simulink model "AutofocusScene"  (R2026a)
settings: Solver=FixedStepDiscrete  StopTime=Cam_SweepTime + Cam_TailTime  FixedStep=Scene_Ts
model workspace (MAT data in the model file):
  AF_CoarseStep = 0.04
  AF_ConfirmTime = 0.25
  AF_FineSpan = 0.04
  AF_FineStep = 0.012
  AF_FocusMax = 30
  AF_FocusMin = 3
  AF_Gain = 0.9
  AF_LevelFloor = 1e-06
  AF_LockThreshold = 0.015
  AF_MaxSlew = 0.08
  AF_MinDwell = 1
  AF_MinSweepSteps = 4
  AF_PeakRatio = 3
  AF_ProbeSize = 0.002
  AF_SearchTrigger = 0.5
  AF_SpotFraction = 0.195
  AF_StopFraction = 0.7
  AF_TopFraction = 0.1
  AF_WinMargin = 1.15
  Cam_FocalLength = [554 554]
  Cam_HandAmount = 1
  Cam_Height = 1.5
  Cam_ImageSize = [480 640]
  Cam_OpticalCenter = [320 240]
  Cam_Pitch = 5
  Cam_SweepTime = 25
  Cam_TailPitch = 10
  Cam_TailTime = 6
  Cam_X = 2.5
  Cam_Y = -2
  Cam_YawStart = -75
  Cam_YawSweep = 100
  Depth_MaxRange = 30
  Scene_Ts = 0.05
undefined symbols (not defined in the file or in its folder): Sim3dSensor
libraries: slpidlib x1, simulink x1, sim3dcameralib x1, sim3dlib x1
settings Model: SimulationMode=accelerator  Creator=csaunder  LastModifiedBy=csaunder
settings DebuggingCC: MergeDetectMultiDrivingBlocksExec=error
settings ModelReferenceCC: PropagateSignalLabelsOutOfModel=on

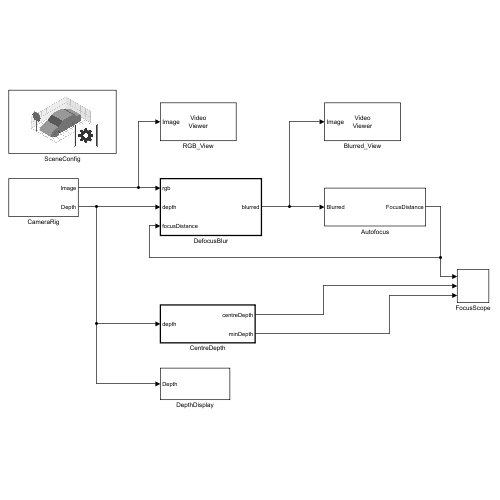
[thumbnail: Simulink's stored preview of the top-level diagram]
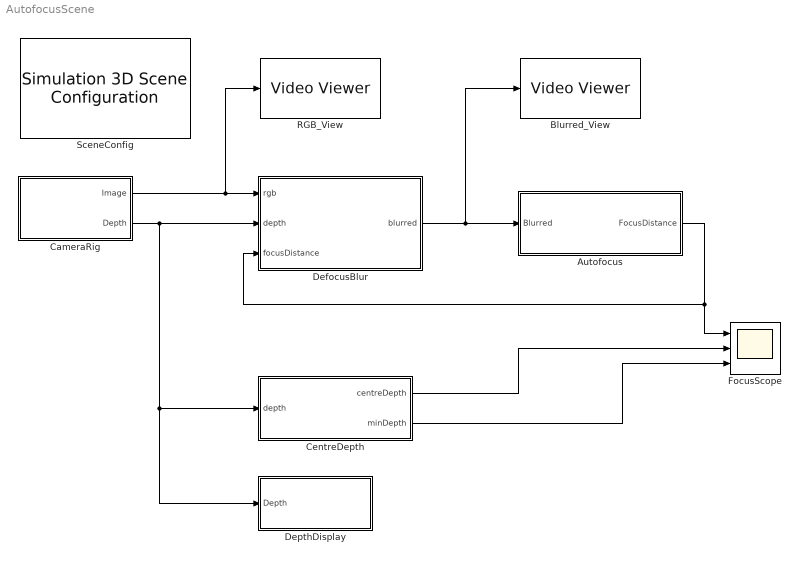
== system AutofocusScene ==
  Autofocus : Subsystem
  Blurred_View : VideoViewer  FigPos=[672 571 507 337]
  CameraRig : Subsystem
  CentreDepth : MATLAB Function  TreatAsAtomicUnit=on
  DefocusBlur : MATLAB Function  TreatAsAtomicUnit=on
  DepthDisplay : Subsystem
  FocusScope : Scope  NumInputPorts=3
  RGB_View : VideoViewer  FigPos=[99 545 418 304]
  SceneConfig : sim3dlib/Simulation 3D Scene Configuration  Priority=0  ProjectFormat=Default Scenes  SceneDesc=Large parking lot  ProjectName=C:\Program Files\MATLAB\R2026a\toolbox\shared\sim3d_projects\automotive_project_windows\UE\WindowsNoEditor\VehicleSimulation.exe  ScenePath=/Game/Maps/HwStrght  EnableOpenDRIVE=off  vehTagList={'Custom';'Scene Origin'}  vehTag=Scene Origin  AttachedCameraRelativeTranslation=[0 0 0]  FreeCameraDefaultInitialTranslation=[-6, 0, 2]  AttachedCameraRelativeRotation=[0, -15, 0]  FreeCameraDefaultInitialRotation=[0, -15, 0]  ViewpointName=Custom  FreeCameraInitialTranslation=[0, 0, 0]  FreeCameraInitialRotation=[0, 0, 0]  OpVisEn=off  Ts=Scene_Ts  EnableWindow=on  EnableRemoteAccess=off  SimulationMode=CoSimulation  SimulateUsing=Interpreted execution  EnableAnimationRecording=off  OverrideDefaultRecording=off  AnimationRecordingFileName=sim3dAnimation.mat  AnimationRecordingInterval=[0 inf]  EnableWeather=off  SunAzimuth=90  SunAltitude=40.0  EnableGeospatialSun=off  Latitude=0  Longitude=0  Date=2023-01-01  Time=10:30:00  GeoTimeZone=-5.0  SunDaylightSaving=off  wind=1  clouds=10  EnableVolumetricClouds=off  CloudCoverage=0  CloudAltitude=6  fog=0  rain=0  RaindropsEffect=off  SnowDensity=0  EnableGeospatial=off  TilesetSource=Earth terrain  UseTrueOrigin=off  OriginHeight=200  OriginLatitude=40.744652  OriginLongitude=-73.988864  MapStyle=Aerial  AdditionalAssetIDs=[]  UseAdvancedSunSky=off  SolarTime=11  TimeZone=-5  Day=21  Month=9  Year=2022  UseDaylightSavingTime=on  DSTStartDay=10  DSTStartMonth=3  DSTEndDay=3  DSTEndMonth=11  DSTSwitchHour=2  sensorTag=MainCamera1  sensorId=1  sensorName=MainCamera1  mountLoc=Origin  offsetFlag=off  tmountOffset=[0, 0, 0]  rmountOffset=[0, 0, 0]  HorizontalResolution=1280  VerticalResolution=720  HorizontalFOV=60  mountPoint=[0 0 0]  mountOrientation=[0 0 0]  aMode=5  ID=1  GeoTrigger=Inactive  ViewNameList={'Custom'}  ViewTranslationList={'[0 0 0]'}  ViewRotationList={'[0 0 0]'}
      link override Simulation 3D Engine: SceneDesc=Large parking lot
      settings: LibrarySourceBlock=sl3dlib/Simulation 3D/Environment/Simulation 3D Scene Configuration
  wires:
  CameraRig/1(Image) -> RGB_View/1, DefocusBlur/1(rgb)
  CameraRig/2(Depth) -> DepthDisplay/1(Depth), CentreDepth/1(depth), DefocusBlur/2(depth)
  DefocusBlur/1(blurred) -> Blurred_View/1, Autofocus/1(Blurred)
  Autofocus/1(FocusDistance) -> FocusScope/1, DefocusBlur/3(focusDistance)
  CentreDepth/1(centreDepth) -> FocusScope/2
  CentreDepth/2(minDepth) -> FocusScope/3

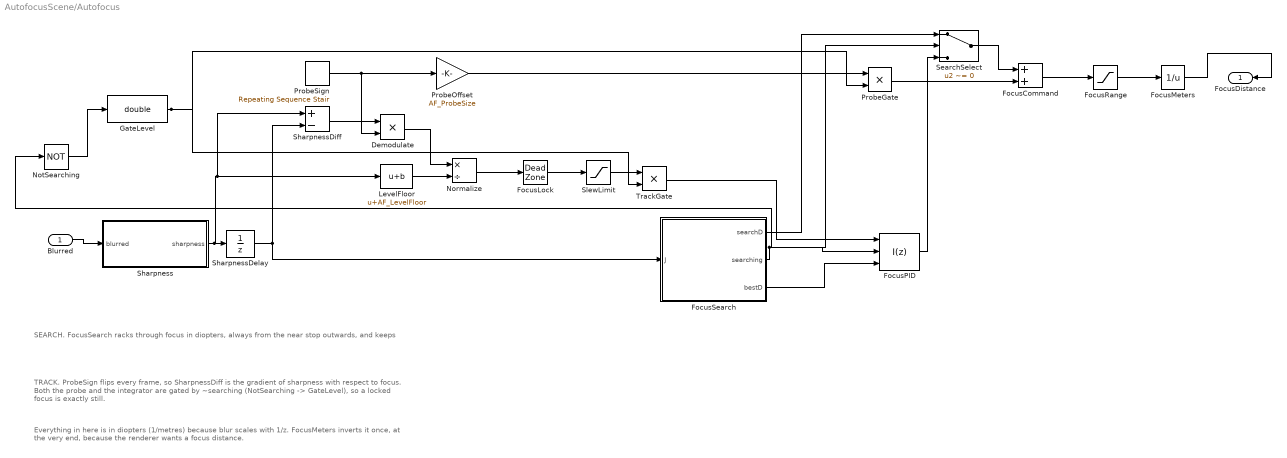
== system AutofocusScene/Autofocus ==
  note: SEARCH. FocusSearch racks through focus in diopters, always from the near stop outwards, and keeps
  note: TRACK. ProbeSign flips every frame, so SharpnessDiff is the gradient of sharpness with respect to focus.
      | Both the probe and the integrator are gated by ~searching (NotSearching -> GateLevel), so a locked focus is exactly still.
  note: Everything in here is in diopters (1/metres) because blur scales with 1/z. FocusMeters inverts it once, at the
      | very end, because the renderer wants a focus distance.
  Blurred : Inport
  Demodulate : Product
  FocusCommand : Sum
  FocusLock : DeadZone  LowerValue=-AF_LockThreshold  UpperValue=AF_LockThreshold
  FocusMeters : Math  Operator=reciprocal
  FocusPID : slpidlib/PID Controller  Controller=I  Form=Parallel  TimeDomain=Discrete-time  UseExternalTs=off  SampleTime=Scene_Ts  IntegratorMethod=Forward Euler  FilterMethod=Forward Euler  ControllerParametersSource=internal  P=1  I=AF_Gain  UseKiTs=off  D=0  UseExternalDerivativeSource=off  N=100  UseFilter=on  TunerSelectOption=Transfer Function Based (PID Tuner App)  InitialConditionSource=external  InitialConditionForIntegrator=1/10  InitialConditionForFilter=0  DifferentiatorICPrevScaledInput=0  ExternalReset=falling  TrackingMode=off  Kt=1  LimitOutput=on  SatLimitsSource=internal  UpperSaturationLimit=1/AF_FocusMin  LowerSaturationLimit=1/AF_FocusMax  LinearizeAsGain=on  AntiWindupMode=clamping  Kb=1  LimitIntegrator=off  UpperIntegratorSaturationLimit=inf  LowerIntegratorSaturationLimit=-inf  POutMin=[]  POutMax=[]  IOutMin=[]  IOutMax=[]  DOutMin=[]  DOutMax=[]  NOutMin=[]  NOutMax=[]  SumOutMin=[]  SumOutMax=[]  SaturationOutMin=[]  SaturationOutMax=[]  PParamMin=[]  PParamMax=[]  IParamMin=[]  IParamMax=[]  DParamMin=[]  DParamMax=[]  NParamMin=[]  NParamMax=[]  KbParamMin=[]  KbParamMax=[]  KtParamMin=[]  KtParamMax=[]  KbOutMin=[]  KbOutMax=[]  KtOutMin=[]  KtOutMax=[]  IntegratorOutMin=[]  IntegratorOutMax=[]  FilterOutMin=[]  FilterOutMax=[]  SumI1OutMin=[]  SumI1OutMax=[]  SumI2OutMin=[]  SumI2OutMax=[]  SumI3OutMin=[]  SumI3OutMax=[]  SumI4OutMin=[]  SumI4OutMax=[]  SumDOutMin=[]  SumDOutMax=[]  DifferentiatorOutMin=[]  DifferentiatorOutMax=[]  FilterDiffOutCoefMin=[]  FilterDiffOutCoefMax=[]  ReciprocalOutMin=[]  ReciprocalOutMax=[]  SumDenOutMin=[]  SumDenOutMax=[]  SumNumOutMin=[]  SumNumOutMax=[]  DivideOutMin=[]  DivideOutMax=[]  UdiffTsProdOutMin=[]  UdiffTsProdOutMax=[]  NTsProdOutMin=[]  NTsProdOutMax=[]  UintegralTsProdOutMin=[]  UintegralTsProdOutMax=[]  UngainTsProdOutMin=[]  UngainTsProdOutMax=[]  ClampingZeroOutDataTypeStr=Inherit: Inherit via back propagation  ClampingZeroOutMin=[]  ClampingZeroOutMax=[]  FilterDenConstantOutDataTypeStr=Inherit: Inherit via back propagation  FilterDenConstantOutMin=[]  FilterDenConstantOutMax=[]  PCopyOutDataTypeStr=Inherit: Inherit via back propagation  PCopyOutMin=[]  PCopyOutMax=[]  NCopyOutDataTypeStr=Inherit: Inherit via back propagation  NCopyOutMin=[]  NCopyOutMax=[]  IntegratorContinuousStateAttributes=''  IntegratorStateMustResolveToSignalObject=off  IntegratorRTWStateStorageClass=Auto  FilterContinuousStateAttributes=''  FilterStateMustResolveToSignalObject=off  FilterRTWStateStorageClass=Auto  ParallelPVariant=Disabled  IdealPVariant=Disabled  IVariant=InternalParameters  DVariant=Disabled  IntegratorVariant=Discrete  SatVariant=Enabled  AWVariant=DiscClampingParallel  PCopyVariant=Disabled  TRVariant=Disabled  FdbkBlocksVariant=Forward  IdealPFdbkVariant=Disabled  SatFdbkVariant=Disabled  DerivativeFilterVariant=Disabled  NVariant=Disabled  NCopyVariant=Disabled_SignalSpec  FilterICVariant=Disabled  IntegratorICVariant=ExternalICs  ExternalResetVariant=ExternalReset  TRSumVariant=Passthrough  SumFdbkVariant=Disabled  SumVariant=Passthrough_I  TsampFilterVariant=InternalTs  TsampNgainVariant=Passthrough  TsampIntegralVariant=Disabled_SignalSpec  ExternalSaturationOutDataTypeStr=Inherit: Same as second input  DerivativeSourceVariant=Disabled  PreIntVariant=InternalPreInt
  FocusRange : Saturate  UpperLimit=1/AF_FocusMin  LowerLimit=1/AF_FocusMax
  FocusSearch : Stateflow chart  TreatAsAtomicUnit=on
  GateLevel : DataTypeConversion  OutDataTypeStr=double  SaturateOnIntegerOverflow=off  RndMeth=Floor
  LevelFloor : Bias  Bias=AF_LevelFloor  SaturateOnIntegerOverflow=off
  Normalize : Product  Inputs=*/
  NotSearching : Logic  Operator=NOT  AllPortsSameDT=off  OutDataTypeStr=boolean
  ProbeGate : Product
  ProbeOffset : Gain  Gain=AF_ProbeSize
  ProbeSign : simulink/Sources/Repeating Sequence Stair  OutValues=[1 -1]  tsamp=Scene_Ts  OutMin=[]  OutMax=[]  OutDataTypeStr=double  OutputDataTypeScalingMode=double  OutDataType=fixdt(0,8)  ConRadixGroup=Best Precision: Vector-wise  OutScaling=2^-12
  SearchSelect : Switch  Criteria=u2 ~= 0  SaturateOnIntegerOverflow=off  InputSameDT=off
  Sharpness : MATLAB Function  TreatAsAtomicUnit=on
  SharpnessDelay : UnitDelay  SampleTime=Scene_Ts
  SharpnessDiff : Sum  Inputs=+-
  SlewLimit : Saturate  UpperLimit=AF_MaxSlew/AF_Gain  LowerLimit=-AF_MaxSlew/AF_Gain
  TrackGate : Product
  FocusDistance : Outport
  wires:
  Blurred/1 -> Sharpness/1(blurred)
  FocusPID/1 -> SearchSelect/3
  Sharpness/1(sharpness) -> LevelFloor/1, SharpnessDiff/1, SharpnessDelay/1
  SharpnessDelay/1 -> SharpnessDiff/2, FocusSearch/1(J)
  Demodulate/1 -> Normalize/1
  ProbeSign/1 -> ProbeOffset/1, Demodulate/2
  SharpnessDiff/1 -> Demodulate/1
  LevelFloor/1 -> Normalize/2
  ProbeOffset/1 -> ProbeGate/1
  Normalize/1 -> FocusLock/1
  FocusLock/1 -> SlewLimit/1
  SlewLimit/1 -> TrackGate/1
  TrackGate/1 -> FocusPID/1
  FocusSearch/1(searchD) -> SearchSelect/1
  FocusSearch/3(bestD) -> FocusPID/3
  ProbeGate/1 -> FocusCommand/2
  SearchSelect/1 -> FocusCommand/1
  FocusCommand/1 -> FocusRange/1
  FocusRange/1 -> FocusMeters/1
  FocusMeters/1 -> FocusDistance/1
  GateLevel/1 -> TrackGate/2, ProbeGate/2
  NotSearching/1 -> GateLevel/1
  FocusSearch/2(searching) -> NotSearching/1, FocusPID/2, SearchSelect/2

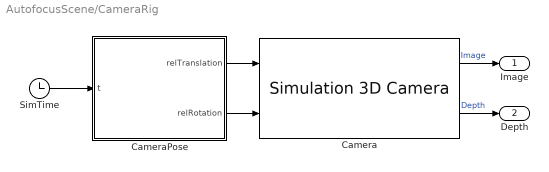
== system AutofocusScene/CameraRig ==
  Camera : sim3dcameralib/Simulation 3D Camera  Priority=1  sensorTag=Sim3dSensor�  sensorId=1  sensorName=Sim3dSensor�  vehTagList={'Scene Origin'}  vehTag=Scene Origin  CoordinateSystem=ISO8855  mountLoc=Origin  offsetFlag=on  tmountOffset=[0, 0, 0]  extTmount=on  rmountOffset=[0, 0, 0]  extRmount=on  FocalLength=Cam_FocalLength  OpticalCenter=Cam_OpticalCenter  ImageSize=Cam_ImageSize  RadialDistortion=[0, 0]  TangentialDistortion=[0, 0]  SensorSkew=0  VisualizeFieldOfView=off  FieldOfViewRange=61  DepthOutportEnabled=on  SemanticOutportEnabled=off  TransformOutportEnabled=off  SampleTime=-1  mountPoint=[0 0 0]  mountOrientation=[0 0 0]  aMode=5  ID=1
      settings: LibrarySourceBlock=sl3dlib/Simulation 3D/Sensors/Simulation 3D Camera
  CameraPose : MATLAB Function  TreatAsAtomicUnit=on
  SimTime : Clock
  Image : Outport
  Depth : Outport  Port=2
  wires:
  Camera/1 -> Image/1  "Image"
  SimTime/1 -> CameraPose/1(t)
  CameraPose/1(relTranslation) -> Camera/1
  CameraPose/2(relRotation) -> Camera/2
  Camera/2 -> Depth/1  "Depth"

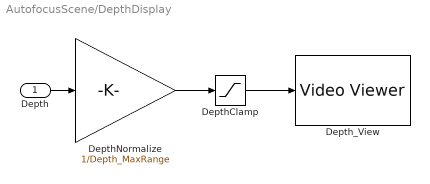
== system AutofocusScene/DepthDisplay ==
  Depth : Inport
  DepthClamp : Saturate  UpperLimit=1  LowerLimit=0
  DepthNormalize : Gain  Gain=1/Depth_MaxRange
  Depth_View : VideoViewer  FigPos=[268 537 418 304]
  wires:
  Depth/1 -> DepthNormalize/1
  DepthNormalize/1 -> DepthClamp/1
  DepthClamp/1 -> Depth_View/1

== matlab function AutofocusScene/DefocusBlur ==
  data: rgb input; blurred output; depth input; focusDistance input
function blurred = DefocusBlur(rgb, depth, focusDistance)
% Defocus the camera image using the thin-lens renderer in simulateDefocusBlur, with
% the optics set in blurSceneImage and the focus plane driven from outside.
%
% The renderer is ordinary MATLAB and is not meant for code generation, so it is
% called extrinsically. An extrinsic call tells Simulink nothing about what comes
% back, which is why blurred is pre-assigned: that fixes its size and class.
coder.extrinsic("blurSceneImage");

blurred = zeros(size(rgb, 1), size(rgb, 2), 3, "uint8");
blurred = blurSceneImage(rgb, depth, focusDistance);
end

== matlab function AutofocusScene/CameraRig/CameraPose ==
  data: t input; relTranslation output; relRotation output; Cam_X parameter; Cam_Y parameter; Cam_Height parameter; Cam_Pitch parameter; Cam_YawStart parameter; Cam_YawSweep parameter; Cam_SweepTime parameter; Cam_HandAmount parameter; Cam_TailTime parameter; Cam_TailPitch parameter
function [relTranslation, relRotation] = CameraPose(t, Cam_X, Cam_Y, Cam_Height, Cam_Pitch, Cam_YawStart, Cam_YawSweep, Cam_SweepTime, Cam_HandAmount, Cam_TailTime, Cam_TailPitch)
%#codegen
% Pan the camera past cars parked at different distances, as if it were being held.
%
% The nominal move is a steady yaw sweep from a fixed spot: the camera does not travel, so
% the distance to the subject changes only because the lens is turning, which is what gives
% the autofocus something to track with only one thing to explain.
%
% On top of that, a hand. Real handheld footage is not a constant rate plus white noise. A
% person's wrist, elbow and breathing each drift at their own slow rate, so the result is a
% few incommensurate sways. Summing sines reproduces that character and, unlike rand, is
% bitwise repeatable from run to run, which matters because every autofocus change here is
% judged by comparing one run against the last. Cam_HandAmount scales all of it, so setting
% it to 0 recovers the original perfectly steady pan.
%
% Coordinate system is ISO8855: X forward, Y left, Z up, translation in m and rotation in
% deg, with positive pitch looking down.

% Progress along the pan, wobbled so the rate is not machine-perfect. The amplitude is
% capped at 0.010 for a reason: d(progress)/dt is 1/Cam_SweepTime - 0.010*2*pi*0.21, which
% stays positive, so the pan slows and quickens between roughly 2.7 and 5.3 deg/s but never
% reverses. A camera that visibly backs up reads as broken rather than as handheld.
%
% Note that progress is NOT clamped at 1. The run is Cam_SweepTime + Cam_TailTime long, so the
% yaw keeps turning through the tail at the same nominal rate, reaching about +49 deg. Dividing
% by Cam_SweepTime rather than by the total is deliberate: it leaves the first Cam_SweepTime
% seconds bit-for-bit identical to every run recorded before the tail existed, so none of the
% earlier A/B comparisons are invalidated by adding it.
progress = t/Cam_SweepTime + Cam_HandAmount*0.010*sin(2*pi*0.21*t);
yaw = Cam_YawStart + Cam_YawSweep*progress;

% The tail ramp, 0 before Cam_SweepTime and 1 at the end of the run. Smoothstep rather than a
% straight line because a linear ramp steps the pitch *rate* discontinuously at the join, which
% reads as a jerk on a camera that is otherwise being held smoothly; 3s^2-2s^3 has zero slope at
% both ends. max() on the denominator keeps Cam_TailTime = 0 from dividing by zero when the tail
% is switched off.
tailFrac = min(max((t - Cam_SweepTime)/max(Cam_TailTime, 1e-6), 0), 1);
tailFrac = tailFrac*tailFrac*(3 - 2*tailFrac);

% Aim drift, in degrees, kept under half a degree in total. At this 60 deg field of view
% that is well under 1% of the frame width, which reads as held-by-a-person rather than
% shaky. Frequencies are deliberately not multiples of each other so the pattern never
% settles into an obvious repeat.
%
% The tail adds Cam_TailPitch of downward tilt on top. Past about +40 deg of yaw the camera is
% looking down the open lot, which is the stretch the 100 deg sweep was cut short to avoid
% because there is nothing textured out there to focus on. Tipping the camera down puts the lot
% surface and its painted markings back in the centre of frame, at roughly
% Cam_Height/tan(Cam_Pitch + Cam_TailPitch) - about 5.6 m, nearer than the cars the pan has been
% tracking, so it also exercises the sweep's preference for the nearest subject it can focus on.
yaw = yaw + Cam_HandAmount*(0.34*sin(2*pi*0.27*t + 0.7) + 0.16*sin(2*pi*0.73*t + 2.1));
pitch = Cam_Pitch + Cam_TailPitch*tailFrac + ...
    Cam_HandAmount*(0.26*sin(2*pi*0.19*t + 1.3) + 0.12*sin(2*pi*0.61*t));
roll = Cam_HandAmount*0.30*sin(2*pi*0.17*t + 2.6);

% Body sway, in metres: a couple of centimetres of shift and a slower vertical drift for
% breathing. This is small on purpose. It has to be felt, not measured - two centimetres
% against subject distances of 4 to 20 m changes the focus the lens needs by under 0.5%,
% so it adds feel without quietly handing the autofocus extra work to do.
x = Cam_X + Cam_HandAmount*0.020*sin(2*pi*0.23*t + 0.4);
y = Cam_Y + Cam_HandAmount*0.025*sin(2*pi*0.31*t + 1.9);
z = Cam_Height + Cam_HandAmount*0.015*sin(2*pi*0.13*t + 0.9);

relTranslation = [x, y, z];
relRotation = [roll, pitch, yaw];
end

== matlab function AutofocusScene/Autofocus/Sharpness ==
  data: blurred input uint8 size=[Cam_ImageSize(1) Cam_ImageSize(2) 3]; sharpness output double size=1; AF_SpotFraction parameter; AF_TopFraction parameter
function sharpness = Sharpness(blurred, AF_SpotFraction, AF_TopFraction)
%#codegen
% Contrast-detect focus metric: gradient energy in the centre spot, divided by brightness
% squared so the loop reacts to focus rather than to exposure.
%
% The energy is the mean of the sharpest AF_TopFraction of the spot's pixels, not the mean of
% all of them, and that choice matters more than it looks. The subject is a parked car, and a
% car is mostly flat paint: a handful of high-contrast features - window frames, wheel arches,
% shadow lines - surrounded by large low-gradient panels. Averaging over the whole spot buries
% those features under the subject's own flat areas, which flattens the sharpness hill the
% controller has to climb. It is worst exactly when a car is entering the spot and covers only
% part of it, because then the flat lot behind it dilutes the signal as well. Taking a high
% percentile instead makes the metric follow the sharpest content actually present, so the
% hill keeps its shape however much of the spot the subject fills.
%
% What this deliberately does NOT fix: the metric still has no notion of which subject
% deserves focus. A sharp background filling most of the spot scores well whether or not
% something nearer has just arrived, so a near subject entering in front of sharp scenery is
% still a separate problem needing subject-change detection.
%
% Changing this does not disturb any tuning downstream. Every threshold in the loop is a
% ratio - J against refJ in the chart, bestJ against minJ within a sweep, and Normalize
% divides by sharpness itself - so the metric may grow by any factor without retuning.

gray = 0.299*double(blurred(:,:,1)) + 0.587*double(blurred(:,:,2)) + 0.114*double(blurred(:,:,3));
[h, w] = size(gray);
rows = (((1:h)' - (h + 1)/2)/h);
cols = (((1:w) - (w + 1)/2)/w);
spot = (abs(rows) <= AF_SpotFraction/2) & (abs(cols) <= AF_SpotFraction/2);

gx = zeros(h, w);
gy = zeros(h, w);
gx(:, 1:w-1) = diff(gray, 1, 2);
gy(1:h-1, :) = diff(gray, 1, 1);

n = sum(spot(:));

% A sentinel of -1 marks the pixels outside the spot, rather than indexing them out with a
% logical, which keeps every array here fixed-size for codegen. Gradient energy is a sum of
% squares and so never negative, so the sentinels sort to the end; cumsum then yields the
% top-k mean using scalar indexing only, with no variable-size array anywhere. Sorting the
% whole frame to rank 6912 spot pixels is wasteful, but it costs well under a millisecond
% against the 280 ms the defocus renderer spends on the same frame.
e = gx(:).^2 + gy(:).^2;
e(~spot(:)) = -1;
sorted = sort(e, 'descend');
k = min(max(round(AF_TopFraction*n), 1), n);
cumulative = cumsum(sorted);
energy = cumulative(k)/k;

brightness = sum(gray(:).*spot(:))/n;
sharpness = energy/(brightness^2 + 1);
end

== matlab function AutofocusScene/CentreDepth ==
  data: depth input; centreDepth output; AF_SpotFraction parameter; minDepth output
function [centreDepth, minDepth] = CentreDepth(depth, AF_SpotFraction)
%#codegen
% Display only. These are the distances the autofocus ought to settle on, so plotting them
% beside the focus command shows whether the loop is tracking. They are deliberately not
% wired into the loop: using them would make this a feedforward system driven by depth
% rather than a contrast-detect autofocus closed through the optics.
%
% Sky comes back as 1000 m, so those pixels are dropped rather than allowed to drag the
% average out to infinity.
%
% Two numbers, because neither alone is a fair reference. The mean is what the spot
% averages, but the sharpness metric peaks where the most TEXTURED content in the spot is
% sharp, not at the mean, so a spot straddling a car and the lot behind it has a mean that
% matches nothing in the picture. The nearest valid surface is the other bound, and for a
% spot aimed at a car it is usually the car.

[h, w] = size(depth);
rows = (((1:h)' - (h + 1)/2)/h);
cols = (((1:w) - (w + 1)/2)/w);
spot = (abs(rows) <= AF_SpotFraction/2) & (abs(cols) <= AF_SpotFraction/2);

valid = spot(:) & (depth(:) < 100);
centreDepth = sum(depth(:).*valid)/max(sum(valid), 1);

% Masking with inf rather than indexing with a logical keeps this fixed-size for codegen.
masked = depth(:);
masked(~valid) = inf;
minDepth = min(masked);
if ~isfinite(minDepth)
    minDepth = centreDepth;
end
end

== stateflow chart AutofocusScene/Autofocus/FocusSearch ==
  settings: updateMethod=DISCRETE  sampleTime=Scene_Ts
  state Coarse
    en:
    % searching also gates the probe and the integrator, outside the chart: the probe is summed onto
    % the command AFTER the sweep picks searchD, so leaving it on would dither every position the
    % sweep evaluates by +/-AF_ProbeSize - the size of the fine step.
    searching = true;
    % Always sweep near to far, so the loop prefers the nearest subject it can focus on. Costs a
    % visible rack back to the near stop at the start of every sweep.
    searchD = 1/AF_FocusMin;
    bestJ = -1;
    minJ = inf;
    bestD = searchD;
    peaked = false;
    nStep = 0;
    du:
    % J was rendered with the previous searchD, so score it before stepping on. AF_WinMargin > 1
    % makes a later - further - peak beat the near one by a clear margin to take the focus.
    if J > AF_WinMargin*bestJ
    bestJ = J;
    bestD = searchD;
    end
    minJ = min(minJ, J);
    % Stop early only once the hill stands clear of the flattest reading this pass, and never in the
    % first few steps. AF_PeakRatio guards the first: the curve's tail varies ~2x on its own, so a
    % bare 'J fell' test trips on the plain. AF_MinSweepSteps guards the second: beside the near
    % stop a dip is indistinguishable from the far side of a hill, and blocking it is what let
    % AF_StopFraction rise from 0.5 to 0.7 with every pick preserved.
    % nStep counts COMPLETED steps, so the floor first admits reading AF_MinSweepSteps + 1.
    if nStep >= AF_MinSweepSteps && bestJ > AF_PeakRatio*minJ && J < AF_StopFraction*bestJ
    peaked = true;
    end
    % Clamp every step: without it the pass walks past the focus stop, where every position renders
    % the same image and the winner is recorded at a distance the lens cannot reach.
    searchD = min(max(searchD - AF_CoarseStep, 1/AF_FocusMax), 1/AF_FocusMin);
    nStep = nStep + 1;
  state Fine
    en:
    coarseD = bestD;
    % Re-enter on the near side of the coarse winner and step outward again, so the near-side
    % preference carries through the fine pass instead of being undone by it.
    searchD = min(max(coarseD + AF_FineSpan, 1/AF_FocusMax), 1/AF_FocusMin);
    bestJ = -1;
    minJ = inf;
    bestD = coarseD;
    peaked = false;
    nStep = 0;
    du:
    if J > AF_WinMargin*bestJ
    bestJ = J;
    bestD = searchD;
    end
    minJ = min(minJ, J);
    % Same three-part early stop as Coarse, step floor included - see the comment there.
    if nStep >= AF_MinSweepSteps && bestJ > AF_PeakRatio*minJ && J < AF_StopFraction*bestJ
    peaked = true;
    end
    searchD = min(max(searchD - AF_FineStep, 1/AF_FocusMax), 1/AF_FocusMin);
    nStep = nStep + 1;
  state Track
    en:
    % What the sweep achieved on THIS content. Only used to decide when to sweep again, never as the
    % tracking reference - tracking needs none.
    refJ = bestJ;
    % Track continuously: not sweeping IS tracking. Holding the lens still is left to FocusLock, the
    % dead zone on the normalised gradient - a differential measurement is immune to scene content
    % drifting through the window, whereas a remembered sharpness level is not. Achievable J swings
    % ~3x with content while the lens sits still, which made the old hysteresis unfixable.
    searching = false;
    dwell = 0;
    stale = false;
    du:
    dwell = dwell + 1;
    % Confirm the sweep's winner briefly before trusting it for a whole AF_MinDwell. A sweep whose
    % readings straddled a change in the spot scored different subjects at different positions and
    % settled on a distance that suits none of them; that shows up within a few frames as J far
    % below the sweep's own bestJ. The window closes so this cannot become a second, permanent
    % re-sweep trigger.
    stale = dwell*Scene_Ts >= AF_ConfirmTime && dwell*Scene_Ts <= 2*AF_ConfirmTime && J < AF_SearchTrigger*refJ;
  (default) -> Coarse
  Coarse -> Fine : [peaked || nStep >= ceil((1/AF_FocusMin - 1/AF_FocusMax)/AF_CoarseStep)]
  Track -> Coarse : [stale || (dwell*Scene_Ts > AF_MinDwell && J < AF_SearchTrigger*refJ)]
  Fine -> Track : [peaked || nStep >= ceil(2*AF_FineSpan/AF_FineStep)]
  data: J input double; searchD output double; searching output boolean; bestD output double; bestJ local double; coarseD local double; dwell local double; AF_FocusMin parameter; AF_FocusMax parameter; AF_CoarseStep parameter; AF_FineStep parameter; AF_FineSpan parameter; AF_SearchTrigger parameter; AF_MinDwell parameter; Scene_Ts parameter; refJ local double; peaked local boolean; nStep local double; AF_StopFraction parameter; minJ local; AF_PeakRatio parameter; AF_WinMargin parameter; AF_ConfirmTime parameter; stale local boolean; AF_MinSweepSteps parameter
